simulink model "sim"  (R2024a)
settings: Solver=VariableStepAuto  StartTime=0.0  StopTime=10.0  RelTol=1e-3
values from neighbouring files (symbols this model uses):
  k_l = (1/2) * ro * C_d * A    (= 0.0405988018623)    [rakett_init.m]
  m = 100    [rakett_init.m]
  r = 0    [rakett_init.m]
settings Model: Creator=Lars André  LastModifiedBy=Lars André

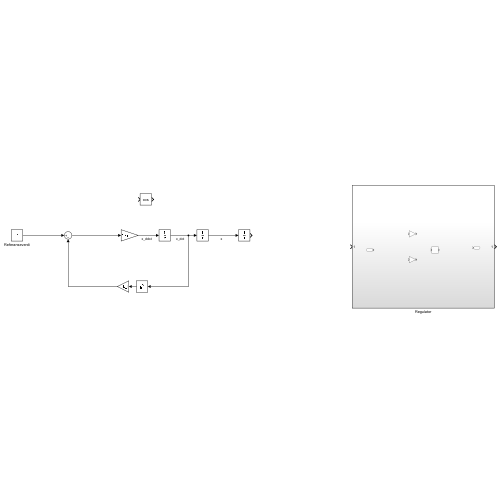
[thumbnail: Simulink's stored preview of the top-level diagram]
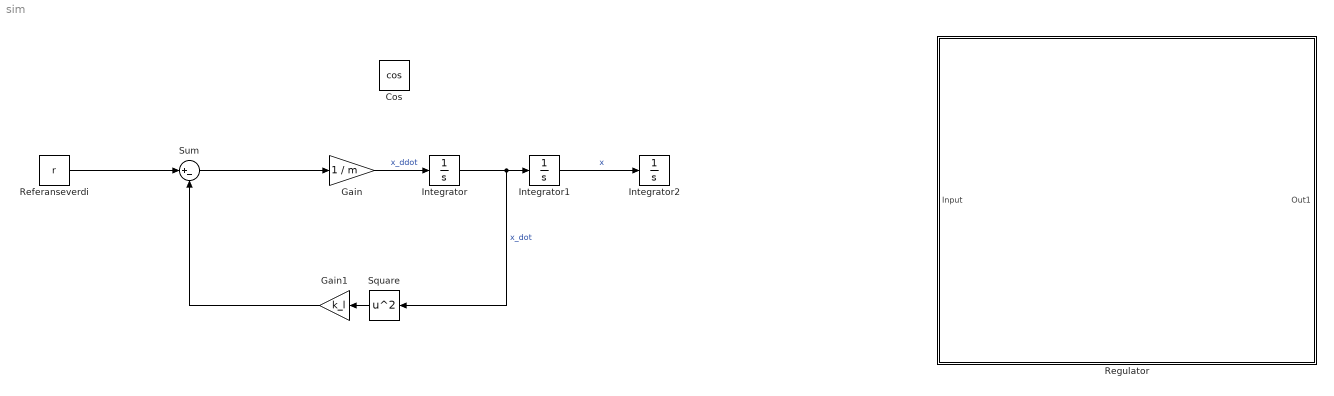
== system sim ==
  Cos : Trigonometry  Operator=cos
  Gain : Gain  Gain=1 / m
  Gain1 : Gain  Gain=k_l
  Integrator : Integrator
  Integrator1 : Integrator
  Integrator2 : Integrator
  Referanseverdi : Constant  Value=r
  Regulator : Subsystem
  Square : Math  Operator=square
  Sum : Sum  Inputs=|+-
  wires:
  Referanseverdi/1 -> Sum/1
  Gain/1 -> Integrator/1  "x_ddot"
  Integrator/1 -> Square/1, Integrator1/1  "x_dot"
  Integrator1/1 -> Integrator2/1  "x"
  Sum/1 -> Gain/1
  Gain1/1 -> Sum/2
  Square/1 -> Gain1/1

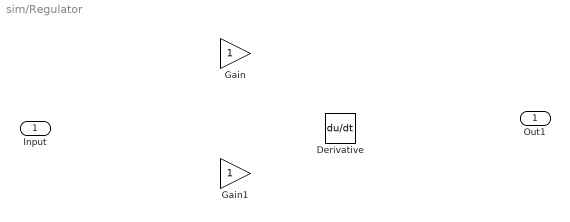
== system sim/Regulator ==
  Input : Inport
  Derivative : Derivative
  Gain : Gain
  Gain1 : Gain
  Out1 : Outport
